simulink model "penduloPID"  (R2015a)
settings: Solver=ode4  StartTime=0.0  StopTime=100.0  FixedStep=0.001  RelTol=1e-3
undefined symbols (not defined in the file): g, k, l, m
settings Model: Creator=Benjamin Nicolas  LastModifiedBy=Benjamin Nicolas
settings SolverCC: ZeroCrossAlgorithm=Adaptive

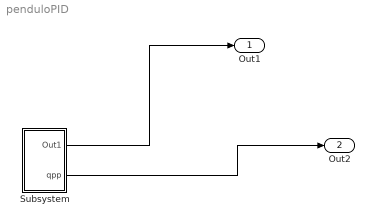
== system penduloPID ==
  Subsystem : Subsystem
  Out1 : Outport
  Out2 : Outport  Port=2
  wires:
  Subsystem/1(Out1) -> Out1/1
  Subsystem/2("qpp ") -> Out2/1

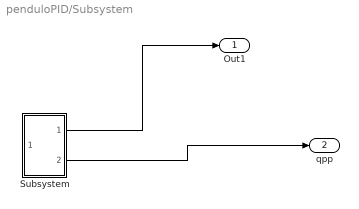
== system penduloPID/Subsystem ==
  Subsystem : Subsystem
  Out1 : Outport
  "qpp " : Outport  Port=2
  wires:
  Subsystem/1(Out1) -> Out1/1
  Subsystem/2("qpp ") -> "qpp "/1

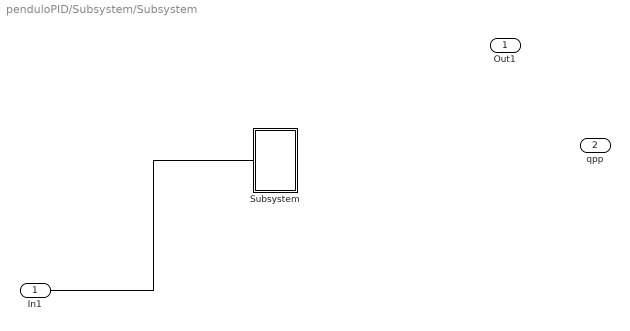
== system penduloPID/Subsystem/Subsystem ==
  In1 : Inport
  Subsystem : Subsystem
  Out1 : Outport
  "qpp " : Outport  Port=2
  wires:
  In1/1 -> ?
  ? -> Out1/1
  ? -> "qpp "/1

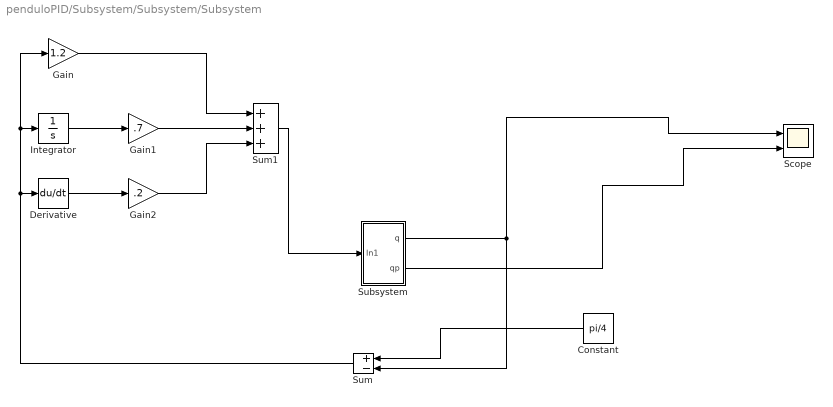
== system penduloPID/Subsystem/Subsystem/Subsystem ==
  Constant : Constant  Value=pi/4
  Derivative : Derivative
  Gain : Gain  Gain=1.2
  Gain1 : Gain  Gain=.7
  Gain2 : Gain  Gain=.2
  Integrator : Integrator
  Scope : Scope  NumInputPorts=2
      settings: YMin=-5~-5  YMax=5~5
  Subsystem : Subsystem
  Sum : Sum  Inputs=+-
  Sum1 : Sum  Inputs=+++
  wires:
  Subsystem/1("q ") -> Sum/2, Scope/1
  Subsystem/2("qp ") -> Scope/2
  Sum1/1 -> Subsystem/1(In1)
  Sum/1 -> Derivative/1, Integrator/1, Gain/1
  Gain/1 -> Sum1/1
  Integrator/1 -> Gain1/1
  Gain1/1 -> Sum1/2
  Derivative/1 -> Gain2/1
  Gain2/1 -> Sum1/3
  Constant/1 -> Sum/1

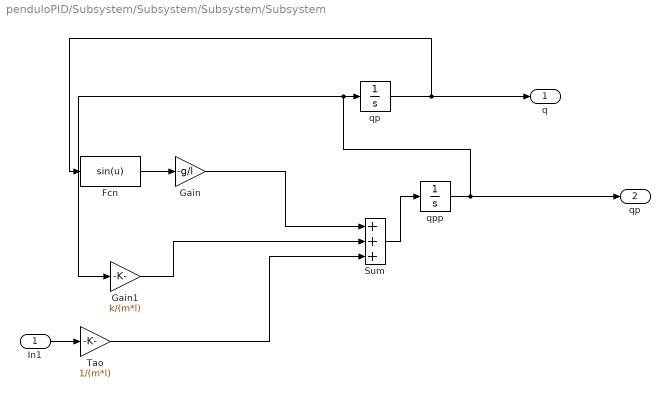
== system penduloPID/Subsystem/Subsystem/Subsystem/Subsystem ==
  In1 : Inport
  Fcn : Fcn  Expr=sin(u)
  Gain : Gain  Gain=-g/l
  Gain1 : Gain  Gain=k/(m*l)
  Sum : Sum  Inputs=+++
  "Tao " : Gain  Gain=1/(m*l)
  qp : Integrator  InitialCondition=pi/2
  qpp : Integrator
  "q " : Outport
  "qp " : Outport  Port=2
  wires:
  Gain1/1 -> Sum/2
  Sum/1 -> qpp/1
  Gain/1 -> Sum/1
  qp/1 -> Fcn/1, "q "/1
  Fcn/1 -> Gain/1
  qpp/1 -> "qp "/1, qp/1, Gain1/1
  In1/1 -> "Tao "/1
  "Tao "/1 -> Sum/3
